simulink model "SCCS_Plant_Model_01"  (R2024a)
settings: Solver=ode3  StartTime=0.0  StopTime=10.0  FixedStep=0.01  RelTol=1e-3
settings Model: Creator=Kishore  LastModifiedBy=Kishore

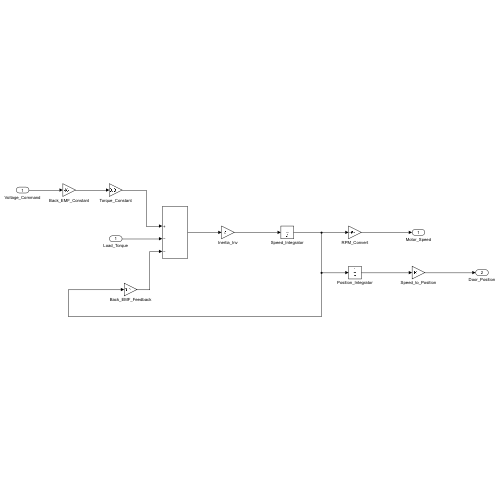
[thumbnail: Simulink's stored preview of the top-level diagram]
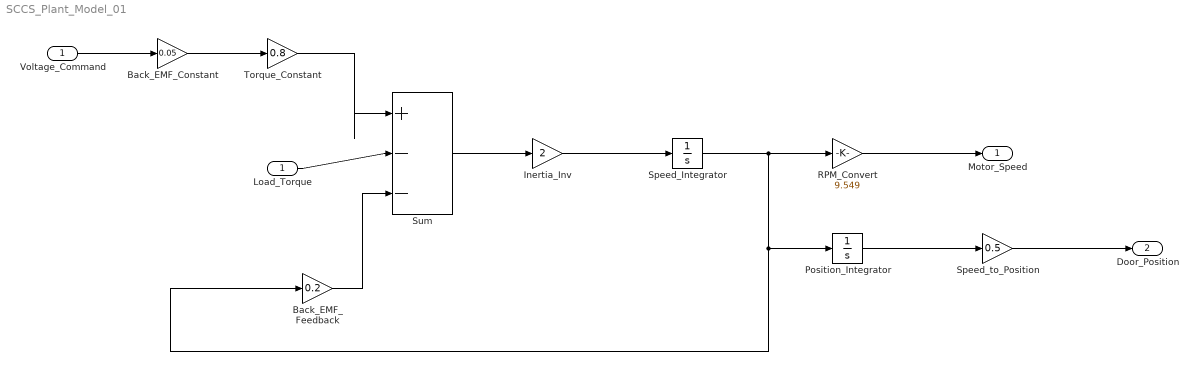
== system SCCS_Plant_Model_01 ==
  Voltage_Command : Inport
  Back_EMF_Constant : Gain  Gain=0.05
  Back_EMF_Feedback : Gain  Gain=0.2
  Inertia_Inv : Gain  Gain=2
  Load_Torque : InportShadow
  Position_Integrator : Integrator
  RPM_Convert : Gain  Gain=9.549
  Speed_Integrator : Integrator
  Speed_to_Position : Gain  Gain=0.5
  Sum : Sum  Inputs=|+--
  Torque_Constant : Gain  Gain=0.8
  Motor_Speed : Outport
  Door_Position : Outport  Port=2
  wires:
  Inertia_Inv/1 -> Speed_Integrator/1
  Speed_Integrator/1 -> RPM_Convert/1, Position_Integrator/1, Back_EMF_Feedback/1
  RPM_Convert/1 -> Motor_Speed/1
  Position_Integrator/1 -> Speed_to_Position/1
  Speed_to_Position/1 -> Door_Position/1
  Back_EMF_Constant/1 -> Torque_Constant/1
  Torque_Constant/1 -> Sum/1
  Sum/1 -> Inertia_Inv/1
  Back_EMF_Feedback/1 -> Sum/3
  Load_Torque/1 -> Sum/2
  Voltage_Command/1 -> Back_EMF_Constant/1
